simulink model "lqr_controller"  (R2024b)
settings: Solver=VariableStepAuto  StartTime=0.0  StopTime=600  RelTol=1e-3
values from neighbouring files (symbols this model uses):
  An = double(subs(Af,{M,m1,m2,l1,l2,g},{1000,100,100,20,10,9.81}))    [PartD_LQRController.m]    (also in PartF_luenberger_observers.m; PartG_LQG_controller.m)
  Bn = double(subs(Bf,{M,m1,m2,l1,l2,g},{1000,100,100,20,10,9.81}))    [PartD_LQRController.m]    (also in PartF_luenberger_observers.m; PartG_LQG_controller.m)
  C = eye(6,6)    [PartB_linearization.m]    (also in PartC_contollability_condition.m; PartD_LQRController.m; PartG_LQG_controller.m = [  0 0 0 0 0 0)
  D = [0;0;0;0;0;0]    [PartB_linearization.m]    (also in PartC_contollability_condition.m; PartD_LQRController.m; PartE_observbliltiy_check.m; PartF_luenberger_observers.m)
  x0 = [0;0;0;0;0.1;-0.1]    [PartB_linearization.m]    (also in PartC_contollability_condition.m = [0;0;0;0;0;0]; PartD_LQRController.m = [0;0;0;5;0;0]; PartE_observbliltiy_check.m = [0;0;0;0;0;0]; PartF_luenberger_observers.m = [0;0;0;0;0;0])
undefined symbols (not defined in the file or in its folder): K

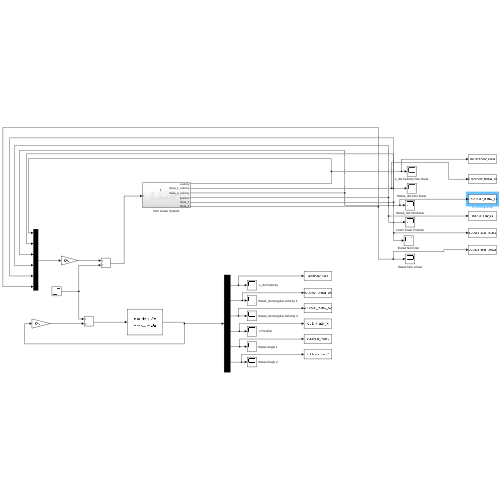
[thumbnail: Simulink's stored preview of the top-level diagram]
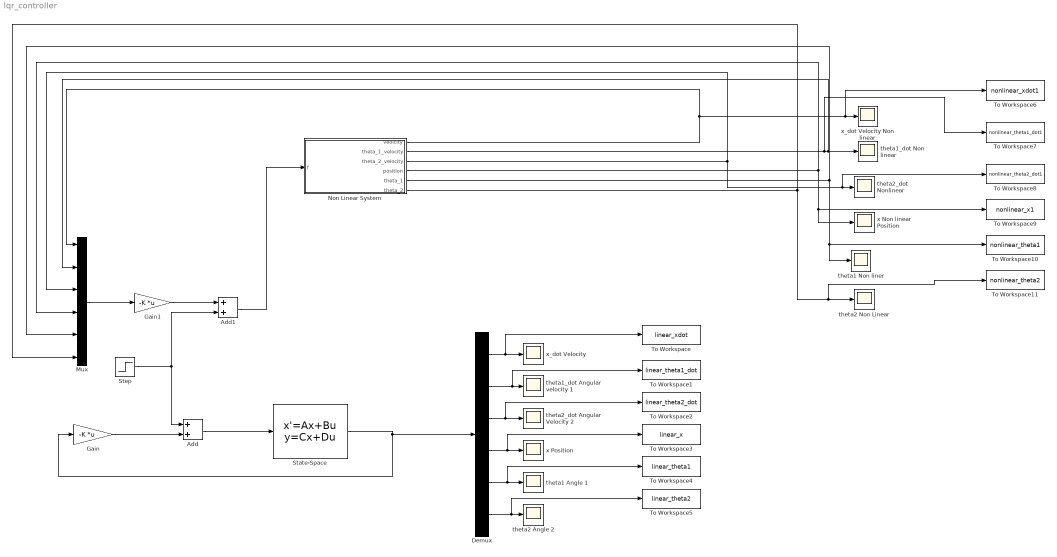
== system lqr_controller ==
  " x Position " : Scope
  " x_dot Velocity" : Scope
  Add : Sum
  Add1 : Sum
  Demux : Demux  Outputs=6
  Gain : Gain  Gain=-K  Multiplication=Matrix(K*u)
  Gain1 : Gain  Gain=-K  Multiplication=Matrix(K*u)
  Mux : Mux  Inputs=6
  Non Linear System : Subsystem
  State-Space : StateSpace  A=An  B=Bn  C=C  D=D  InitialCondition=x0
  Step : Step  After=5000  SampleTime=0
  To Workspace : ToWorkspace  VariableName=linear_xdot  SaveFormat=Timeseries  SampleTime=-1
  To Workspace1 : ToWorkspace  VariableName=linear_theta1_dot  SaveFormat=Timeseries  SampleTime=-1
  To Workspace10 : ToWorkspace  VariableName=nonlinear_theta1  SaveFormat=Timeseries  SampleTime=-1
  To Workspace11 : ToWorkspace  VariableName=nonlinear_theta2  SaveFormat=Timeseries  SampleTime=-1
  To Workspace2 : ToWorkspace  VariableName=linear_theta2_dot  SaveFormat=Timeseries  SampleTime=-1
  To Workspace3 : ToWorkspace  VariableName=linear_x  SaveFormat=Timeseries  SampleTime=-1
  To Workspace4 : ToWorkspace  VariableName=linear_theta1  SaveFormat=Timeseries  SampleTime=-1
  To Workspace5 : ToWorkspace  VariableName=linear_theta2  SaveFormat=Timeseries  SampleTime=-1
  To Workspace6 : ToWorkspace  VariableName=nonlinear_xdot1  SaveFormat=Timeseries  SampleTime=-1
  To Workspace7 : ToWorkspace  VariableName=nonlinear_theta1_dot1  SaveFormat=Timeseries  SampleTime=-1
  To Workspace8 : ToWorkspace  VariableName=nonlinear_theta2_dot1  SaveFormat=Timeseries  SampleTime=-1
  To Workspace9 : ToWorkspace  VariableName=nonlinear_x1  SaveFormat=Timeseries  SampleTime=-1
  theta1 Angle 1 : Scope
  theta1 Non liner : Scope
  "theta1_dot Angular velocity 1 " : Scope
  theta1_dot Non linear : Scope
  theta2 Angle 2 : Scope
  theta2 Non Linear : Scope
  theta2_dot Angular Velocity 2 : Scope
  theta2_dot Nonlinear : Scope
  x Non linear Position : Scope
  x_dot Velocity Non linear : Scope
  wires:
  State-Space/1 -> Demux/1, Gain/1
  Demux/1 -> To Workspace/1, " x_dot Velocity"/1
  Demux/2 -> To Workspace1/1, "theta1_dot Angular velocity 1 "/1
  Demux/3 -> To Workspace2/1, theta2_dot Angular Velocity 2/1
  Demux/4 -> To Workspace3/1, " x Position "/1
  Demux/5 -> To Workspace4/1, theta1 Angle 1/1
  Demux/6 -> To Workspace5/1, theta2 Angle 2/1
  Add/1 -> State-Space/1
  Gain/1 -> Add/2
  Mux/1 -> Gain1/1
  Gain1/1 -> Add1/1
  Step/1 -> Add/1, Add1/2
  Non Linear System/4(position) -> x Non linear Position/1, To Workspace9/1, Mux/4
  Non Linear System/1(veolcity) -> Mux/1, To Workspace6/1, x_dot Velocity Non linear/1
  Non Linear System/5(theta_1) -> To Workspace10/1, theta1 Non liner/1, Mux/5
  Non Linear System/6(theta_2) -> To Workspace11/1, theta2 Non Linear/1, Mux/6
  Non Linear System/2(theta_1_velocity) -> theta1_dot Non linear/1, Mux/2, To Workspace7/1
  Non Linear System/3(theta_2_velocity) -> theta2_dot Nonlinear/1, To Workspace8/1, Mux/3
  Add1/1 -> Non Linear System/1(f)

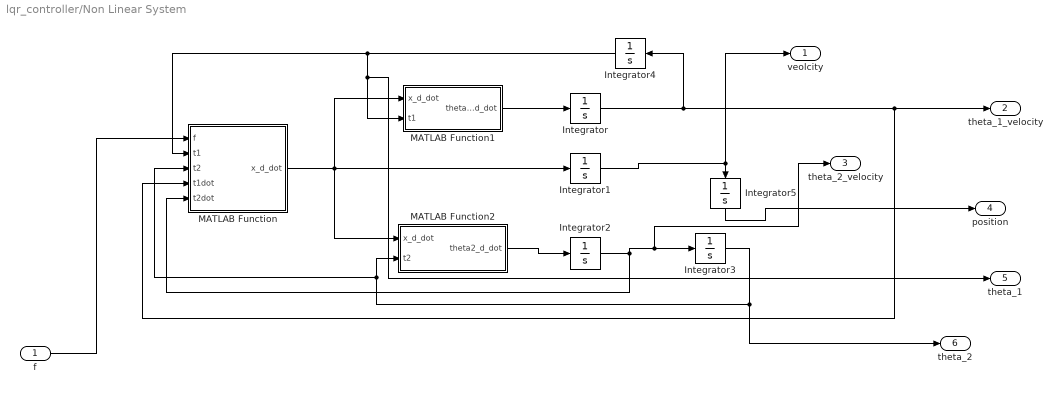
== system lqr_controller/Non Linear System ==
  f : Inport
  Integrator : Integrator  InitialCondition=x0(2)
  Integrator1 : Integrator  InitialCondition=x0(1)
  Integrator2 : Integrator  InitialCondition=x0(3)
  Integrator3 : Integrator  InitialCondition=x0(6)
  Integrator4 : Integrator  InitialCondition=x0(5)
  Integrator5 : Integrator  InitialCondition=x0(4)
  MATLAB Function : MATLAB Function  TreatAsAtomicUnit=on
  MATLAB Function1 : MATLAB Function  TreatAsAtomicUnit=on
  MATLAB Function2 : MATLAB Function  TreatAsAtomicUnit=on
  veolcity : Outport
  theta_1_velocity : Outport  Port=2
  theta_2_velocity : Outport  Port=3
  position : Outport  Port=4
  theta_1 : Outport  Port=5
  theta_2 : Outport  Port=6
  wires:
  f/1 -> MATLAB Function/1(f)
  MATLAB Function2/1(theta2_d_dot) -> Integrator2/1
  MATLAB Function1/1(theta1_d_dot) -> Integrator/1
  Integrator5/1 -> position/1
  Integrator1/1 -> veolcity/1, Integrator5/1
  Integrator2/1 -> theta_2_velocity/1, Integrator3/1, MATLAB Function/5(t2dot)
  Integrator/1 -> Integrator4/1, theta_1_velocity/1, MATLAB Function/4(t1dot)
  Integrator4/1 -> theta_1/1, MATLAB Function1/2(t1), MATLAB Function/2(t1)
  MATLAB Function/1(x_d_dot) -> Integrator1/1, MATLAB Function1/1(x_d_dot), MATLAB Function2/1(x_d_dot)
  Integrator3/1 -> theta_2/1, MATLAB Function/3(t2), MATLAB Function2/2(t2)

== matlab function lqr_controller/Non Linear System/MATLAB Function1 ==
  data: x_d_dot input; theta1_d_dot output; t1 input
function theta1_d_dot = fcn(x_d_dot,t1)

l1 = 20;
theta1_d_dot = (cos(t1)*x_d_dot - 9.81*sin(t1))/l1;

== matlab function lqr_controller/Non Linear System/MATLAB Function ==
  data: f input; x_d_dot output; t1 input; t2 input; t1dot input; t2dot input
function x_d_dot = fcn(f,t1,t2,t1dot,t2dot)

M = 1000;
m1 = 100;
m2 = 100;
g = 9.81;
l1 = 20;
l2 = 10;

x_d_dot = (f - m1*l1*sin(t1)*t1dot^2 -m2*l2*sin(t2)*t2dot^2 -m1*g*sin(t1)*cos(t1) - m2*g*sin(t2)*cos(t2))/(M + m1*(sin(t1))^2 + m2*(sin(t2))^2);

== matlab function lqr_controller/Non Linear System/MATLAB Function2 ==
  data: x_d_dot input; theta2_d_dot output; t2 input
function theta2_d_dot = fcn(x_d_dot,t2)

l2 = 10;
theta2_d_dot = (cos(t2)*x_d_dot - 9.81*sin(t2))/l2;
